simulink library "INT_AFST_VD"  (R2016b)
settings: Solver=VariableStepAuto  StartTime=0.0  StopTime=10.0  RelTol=1e-3
settings Model: Creator=bianxuyin  LastModifiedBy=bianxuyin

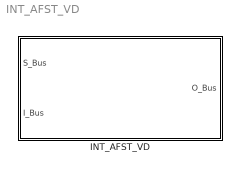
== system INT_AFST_VD ==
  INT_AFST_VD : Subsystem

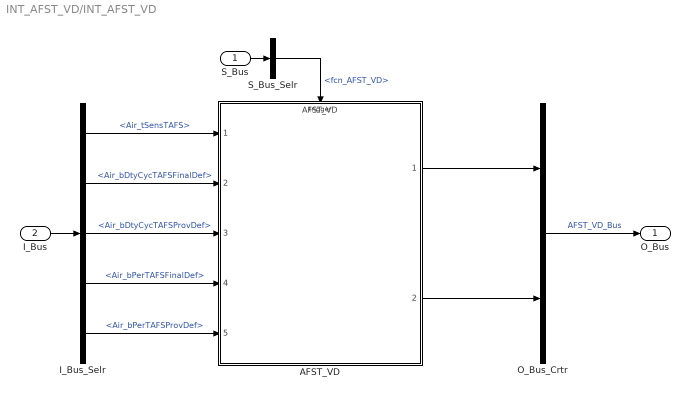
== system INT_AFST_VD/INT_AFST_VD ==
  S_Bus : Inport
  I_Bus : Inport  Port=2
  AFST_VD : ModelReference  ModelNameDialog=AFST_VD  SimulationMode=Normal  ModelReferenceVersion=1.25  TriggerPortName=function  TriggerPortTriggerType=function-call  TriggerPortStatesWhenEnabling=held
  I_Bus_Selr : BusSelector  OutputSignals=Air_tSensTAFS,Air_bDtyCycTAFSFinalDef,Air_bDtyCycTAFSProvDef,Air_bPerTAFSFinalDef,Air_bPerTAFSProvDef
  O_Bus_Crtr : BusCreator  Inputs=2
  S_Bus_Selr : BusSelector  OutputSignals=fcn_AFST_VD
  O_Bus : Outport
  wires:
  S_Bus_Selr/1 -> AFST_VD/Trigger  "<fcn_AFST_VD>"
  S_Bus/1 -> S_Bus_Selr/1
  I_Bus/1 -> I_Bus_Selr/1
  I_Bus_Selr/1 -> AFST_VD/1  "<Air_tSensTAFS>"
  I_Bus_Selr/2 -> AFST_VD/2  "<Air_bDtyCycTAFSFinalDef>"
  I_Bus_Selr/3 -> AFST_VD/3  "<Air_bDtyCycTAFSProvDef>"
  I_Bus_Selr/4 -> AFST_VD/4  "<Air_bPerTAFSFinalDef>"
  I_Bus_Selr/5 -> AFST_VD/5  "<Air_bPerTAFSProvDef>"
  O_Bus_Crtr/1 -> O_Bus/1  "AFST_VD_Bus"
  AFST_VD/1 -> O_Bus_Crtr/1
  AFST_VD/2 -> O_Bus_Crtr/2
